simulink model "DAB_Data_Generate_v2"  (R2021b)
settings: Solver=FixedStepAuto  StartTime=0.0  StopTime=1  FixedStep=1e-6  MaxStep=1e-4  RelTol=1e-3
values from neighbouring files (symbols this model uses):
  f = 50e3    (= 50000)    [DAB_Data_Generation.m]
  N_pri = 1000    [DAB_Data_Generation.m]
  N_sec = 1000    [DAB_Data_Generation.m]
  Vin = 400    [DAB_Data_Generation.m]
undefined symbols (not defined in the file or in its folder): D0, D1, D2, P
libraries: spsOnDelayLib x8, spsIGBTDiodeLib x8, spsVoltageMeasurementLib x4, spsCurrentMeasurementLib x4, spsSeriesRLCBranchLib x3, spsDCVoltageSourceLib x1, spsLinearTransformerLib x1, spsMeanLib x1, spsRMSLib x1, spspowerguiLib x1
settings Model: Creator=mluser  LastModifiedBy=varat
settings SolverCC: AlgebraicLoopSolver=TrustRegion
settings DebuggingCC: ArithmeticOperatorsInVariantConditions=warning
settings SFSimCC: CustomCodeUndefinedFunction=UseInterfaceOnly

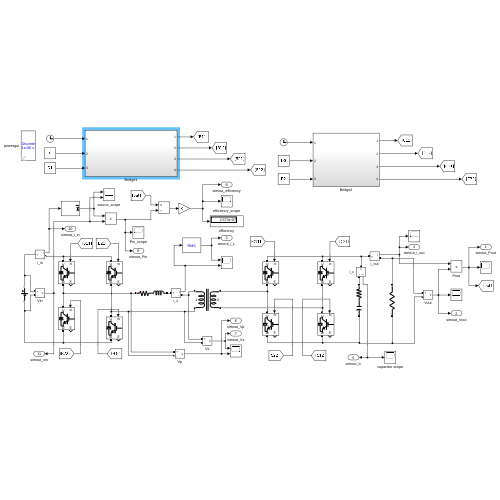
[thumbnail: Simulink's stored preview of the top-level diagram]
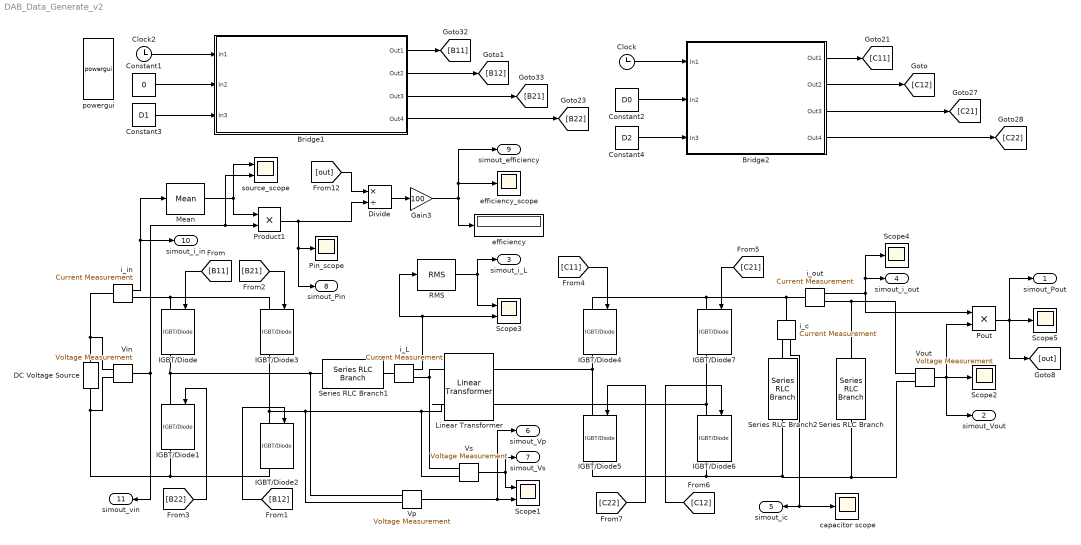
== system DAB_Data_Generate_v2 ==
  Bridge1 : Subsystem
  Bridge2 : Subsystem
  Clock : Clock
  Clock2 : Clock
  Constant1 : Constant  Value=0
  Constant2 : Constant  Value=D0
  Constant3 : Constant  Value=D1
  Constant4 : Constant  Value=D2
  DC Voltage Source : spsDCVoltageSourceLib/DC Voltage Source  Amplitude=Vin  Measurements=None
  Divide : Product  Inputs=*/
  Gain3 : Gain  Gain=100
  IGBT/Diode{,1..7} (8 alike) : spsIGBTDiodeLib/IGBT//Diode  Ron=1e-4  Rs=1e5  Cs=inf  Measurements=on
  Linear Transformer : spsLinearTransformerLib/Linear Transformer  UNITS=SI  NominalPower=[300e3 50000 ]  winding1=[N_pri 0 0]  winding2=[N_sec 0 0]  ThreeWindings=off  winding3=[3.15e+05 793.8 0.10107]  RmLm=[2e+12 3.9789e+08]  Measurements=None  DataType=on
  Mean : spsMeanLib/Mean  Freq=50000  Vinit=0  Ts=0
  Pin_scope : Scope
  Pout : Product
  Product1 : Product
  RMS : spsRMSLib/RMS  TrueRMS=on  Freq=50000  RMSInit=0  Ts=0
  Scope1 : Scope  NumInputPorts=2
  Scope2 : Scope
  Scope3 : Scope  NumInputPorts=2
  Scope4 : Scope
  Scope5 : Scope
  Series RLC Branch : spsSeriesRLCBranchLib/Series RLC Branch  LConnTagsString=__new0  RConnTagsString=__new0  BranchType=R  Resistance=(400*400)/P  Inductance=1e-3  SetiL0=off  InitialCurrent=0  Capacitance=1e-6  Setx0=off  InitialVoltage=0  Measurements=None
  Series RLC Branch1 : spsSeriesRLCBranchLib/Series RLC Branch  LConnTagsString=__new0  RConnTagsString=__new0  BranchType=RL  Resistance=0  Inductance=2.42649e-6  SetiL0=off  InitialCurrent=0  Capacitance=1e-6  Setx0=off  InitialVoltage=0  Measurements=None
  Series RLC Branch2 : spsSeriesRLCBranchLib/Series RLC Branch  LConnTagsString=__new0  RConnTagsString=__new0  BranchType=RC  Resistance=0  Inductance=1e-3  SetiL0=off  InitialCurrent=0  Capacitance=10e-3  Setx0=off  InitialVoltage=0  Measurements=None
  Vin : spsVoltageMeasurementLib/Voltage Measurement  PhasorSimulation=off  OutputType=Complex  PSBequivalent=0
  Vout : spsVoltageMeasurementLib/Voltage Measurement  PhasorSimulation=off  OutputType=Complex  PSBequivalent=0
  Vp : spsVoltageMeasurementLib/Voltage Measurement  PhasorSimulation=off  OutputType=Complex  PSBequivalent=0
  Vs : spsVoltageMeasurementLib/Voltage Measurement  PhasorSimulation=off  OutputType=Complex  PSBequivalent=0
  capacitor scope : Scope
  efficiency : Display
  efficiency_scope : Scope
  i_L : spsCurrentMeasurementLib/Current Measurement  PhasorSimulation=off  OutputType=Complex  PSBequivalent=0
  i_c : spsCurrentMeasurementLib/Current Measurement  PhasorSimulation=off  OutputType=Complex  PSBequivalent=0
  i_in : spsCurrentMeasurementLib/Current Measurement  PhasorSimulation=off  OutputType=Complex  PSBequivalent=0
  i_out : spsCurrentMeasurementLib/Current Measurement  PhasorSimulation=off  OutputType=Complex  PSBequivalent=0
  powergui : spspowerguiLib/powergui  Priority=1  SimulationMode=Discrete  SampleTime=1e-6  frequency=60  Iterations=50  frequencyindice=0  Pbase=100e6  ErrMax=1e-4  UnitsV=kV  UnitsW=MW  buscounter=0  FunctionMessages=off  echomessages=off  EnableUseOfTLC=off  CurrentSourceSwitches=off  DisableSnubberDevices=off  DisableRonSwitches=off  DisableVfSwitches=off  DisplayEquations=off  AutomaticDiscreteSolvers=off  SolverType=Tustin/Backward Euler (TBE)  Interpol=off  ExternalGateDelay=off  methode=off  Ts=100  x0status=blocks  SPID=off  SwTol=0  HookPort=off  NonlinearTolerance=1e-4  nMaxIteration=100  ContinueOnMaxIteration=off  RestoreLinks=warning  ResistiveCurrentMeasurement=off  Frange=[0:2:500]  Ylog=off  Xlog=on  ShowGrid=off  save=off  variable=ZData  structure=0  ZoomFFT=off  StartTime=0.0  cycles=1  DisplayStyle=1  fundamental=60  FreqAxis=off  MaxFrequency=1000  frequencyindicesteady=1  RmsSteady=1  display=off
  source_scope : Scope  NumInputPorts=2
  simout_Pout : Outport
  simout_Vout : Outport  Port=2
  simout_i_L : Outport  Port=3
  simout_i_out : Outport  Port=4
  simout_ic : Outport  Port=5
  simout_Vp : Outport  Port=6
  simout_Vs : Outport  Port=7
  simout_Pin : Outport  Port=8
  simout_efficiency : Outport  Port=9
  simout_i_in : Outport  Port=10
  simout_vin : Outport  Port=11
  wires:
  RMS/1 -> simout_i_L/1, Scope3/1
  [C12] -> IGBT/Diode6/1
  Vin/1 -> simout_vin/1, source_scope/2, Product1/2
  [C11] -> IGBT/Diode4/1
  [B11] -> IGBT/Diode/1
  Mean/1 -> source_scope/1, Product1/1
  [C21] -> IGBT/Diode7/1
  [out] -> Divide/1
  [B21] -> IGBT/Diode3/1
  [B22] -> IGBT/Diode1/1
  [C22] -> IGBT/Diode5/1
  Gain3/1 -> simout_efficiency/1, efficiency_scope/1, efficiency/1
  Product1/1 -> simout_Pin/1, Pin_scope/1, Divide/2
  i_out/1 -> Scope4/1, simout_i_out/1, Pout/1
  Vout/1 -> simout_Vout/1, Scope2/1, Pout/2
  Divide/1 -> Gain3/1
  Pout/1 -> simout_Pout/1, [out], Scope5/1
  i_L/1 -> Scope3/2, RMS/1
  [B12] -> IGBT/Diode2/1
  Bridge2/1(Out1) -> [C11]
  Constant1/1 -> Bridge1/2(In2)
  Clock2/1 -> Bridge1/1(In1)
  Constant2/1 -> Bridge2/2(In2)
  Bridge1/3(Out3) -> [B21]
  Clock/1 -> Bridge2/1(In1)
  Bridge2/4(Out4) -> [C22]
  Bridge1/2(Out2) -> [B12]
  Bridge2/3(Out3) -> [C21]
  Bridge1/1(Out1) -> [B11]
  Bridge2/2(Out2) -> [C12]
  Bridge1/4(Out4) -> [B22]
  Constant4/1 -> Bridge2/3(In3)
  Constant3/1 -> Bridge1/3(In3)
  Vs/1 -> Scope1/1, simout_Vs/1
  Vp/1 -> simout_Vp/1, Scope1/2
  i_c/1 -> simout_ic/1, capacitor scope/1
  i_in/1 -> simout_i_in/1, Mean/1
  connections:
  Vp/LConn1 -- Series RLC Branch1/LConn1 -- IGBT/Diode1/LConn1 -- IGBT/Diode/RConn1
  Linear Transformer/LConn1 -- Vs/LConn1 -- i_L/RConn1
  Vp/LConn2 -- Vs/LConn2 -- Linear Transformer/LConn2 -- IGBT/Diode3/RConn1 -- IGBT/Diode2/LConn1
  i_out/RConn1 -- Vout/LConn1 -- Series RLC Branch/LConn1
  Linear Transformer/RConn1 -- IGBT/Diode5/LConn1 -- IGBT/Diode4/RConn1
  IGBT/Diode5/RConn1 -- IGBT/Diode6/RConn1 -- Series RLC Branch2/RConn1 -- Vout/LConn2 -- Series RLC Branch/RConn1
  i_in/RConn1 -- IGBT/Diode3/LConn1 -- IGBT/Diode/LConn1
  i_out/LConn1 -- IGBT/Diode4/LConn1 -- IGBT/Diode7/LConn1 -- i_c/LConn1
  Linear Transformer/RConn2 -- IGBT/Diode7/RConn1 -- IGBT/Diode6/LConn1
  IGBT/Diode2/RConn1 -- IGBT/Diode1/RConn1 -- Vin/LConn2 -- DC Voltage Source/LConn1
  i_in/LConn1 -- Vin/LConn1 -- DC Voltage Source/RConn1
  i_L/LConn1 -- Series RLC Branch1/RConn1
  Series RLC Branch2/LConn1 -- i_c/RConn1

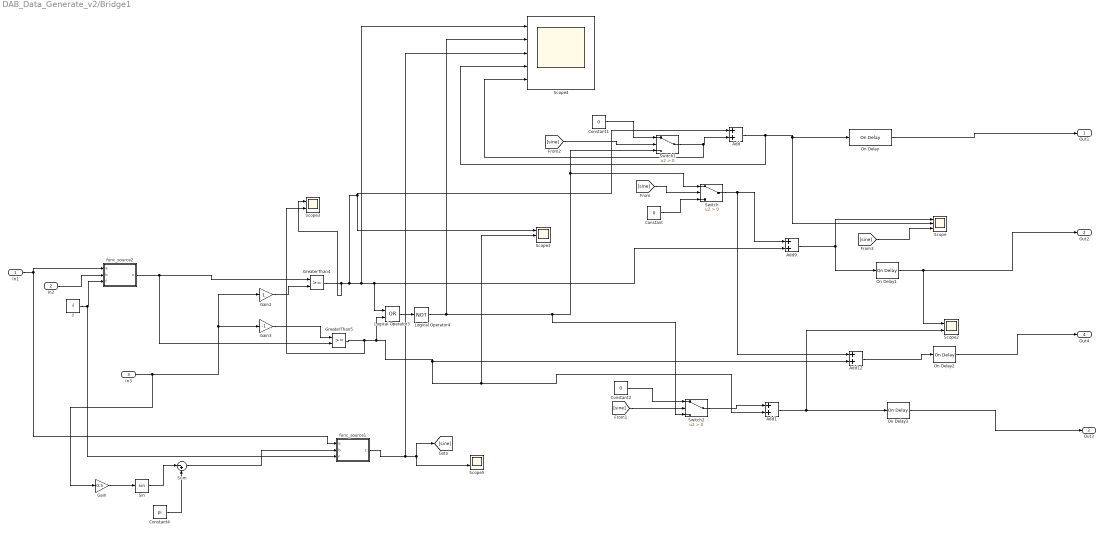
== system DAB_Data_Generate_v2/Bridge1 ==
  In1 : Inport
  In2 : Inport  Port=2
  In3 : Inport  Port=3
  Add{,1,9,12} (4 alike) : Sum
  Constant : Constant  Value=0
  Constant1 : Constant  Value=0
  Constant2 : Constant  Value=0
  Constant4 : Constant  Value=pi
  Gain : Gain  Gain=0.5
  Gain2 : Gain
  Gain3 : Gain  Gain=-1
  GreaterThan4 : RelationalOperator  OutDataTypeStr=boolean  RndMeth=Simplest
  GreaterThan5 : RelationalOperator  OutDataTypeStr=boolean  RndMeth=Simplest
  Logical Operator3 : Logic  Operator=OR  AllPortsSameDT=off  OutDataTypeStr=boolean
  Logical Operator4 : Logic  Operator=NOT  AllPortsSameDT=off  OutDataTypeStr=boolean
  On Delay{,1..3} (4 alike) : spsOnDelayLib/On Delay  DelayType=On delay  delay=0  ic=0  Ts=0
      settings: SourceProductBaseCode=PS
  Scope : Scope  NumInputPorts=3
  Scope1 : Scope  NumInputPorts=3
  Scope2 : Scope  NumInputPorts=2
  Scope3 : Scope  NumInputPorts=2
  Scope4 : Scope  NumInputPorts=5
  Scope5 : Scope  NumInputPorts=2
  Sin : Trigonometry
  Sum : Sum  Inputs=|-+
  Switch : Switch  Criteria=u2 > Threshold
  Switch1 : Switch  Criteria=u2 > Threshold
  Switch2 : Switch  Criteria=u2 > Threshold
  f : Constant  Value=f
  func_source1 : MATLAB Function  TreatAsAtomicUnit=on
  func_source2 : MATLAB Function  TreatAsAtomicUnit=on
  Out1 : Outport  VectorParamsAs1DForOutWhenUnconnected=off
  Out2 : Outport  Port=2  VectorParamsAs1DForOutWhenUnconnected=off
  Out3 : Outport  Port=3  VectorParamsAs1DForOutWhenUnconnected=off
  Out4 : Outport  Port=4  VectorParamsAs1DForOutWhenUnconnected=off
  wires:
  [sine] -> Scope/3
  Gain2/1 -> GreaterThan4/2
  Add/1 -> Scope4/4, Scope/2, On Delay/1
  Add1/1 -> Scope2/2, On Delay3/1
  Add9/1 -> On Delay1/1, Scope/1
  On Delay/1 -> Out1/1
  Add12/1 -> On Delay2/1
  Switch/1 -> Add12/1, Add9/1
  Logical Operator3/1 -> Logical Operator4/1
  Switch2/1 -> Add1/1
  [sine] -> Switch/2
  [sine] -> Switch1/2
  GreaterThan5/1 -> Scope3/2, Scope1/2, Add1/2, Add12/2, Logical Operator3/2
  Logical Operator4/1 -> Scope4/2, Switch2/3, Switch/1, Switch1/3
  Gain3/1 -> GreaterThan5/1
  In3/1 -> Gain/1, Gain3/1, Gain2/1
  [sine] -> Switch2/2
  On Delay3/1 -> Out3/1
  On Delay2/1 -> Out4/1
  On Delay1/1 -> Out2/1, Scope2/1
  GreaterThan4/1 -> Scope3/1, Add/1, Scope1/1, Scope4/1, Add9/2, Logical Operator3/1
  In1/1 -> func_source1/1(a), func_source2/1(a)
  Switch1/1 -> Scope4/5, Add/2
  func_source1/1(z) -> Scope4/3, [sine], Scope5/2
  Sum/1 -> func_source1/2(b)
  func_source2/1(z) -> GreaterThan5/2, GreaterThan4/1
  In2/1 -> func_source2/2(b)
  Constant1/1 -> Switch1/1
  Constant/1 -> Switch/3
  Constant2/1 -> Switch2/1
  Gain/1 -> Sin/1
  Constant4/1 -> Sum/2
  Sin/1 -> Sum/1
  f/1 -> func_source1/3(f), func_source2/3(f)

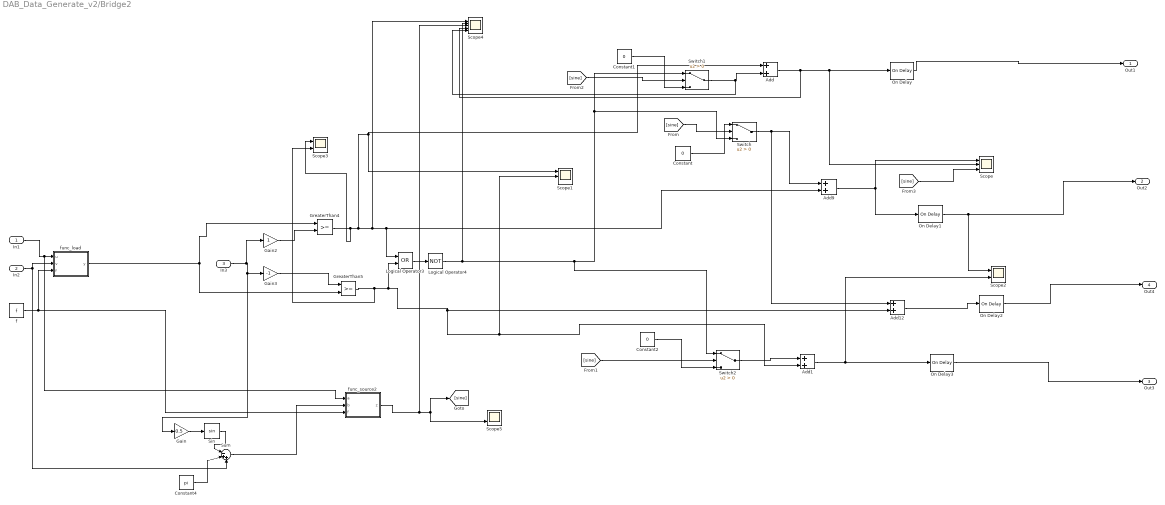
== system DAB_Data_Generate_v2/Bridge2 ==
  In1 : Inport
  In2 : Inport  Port=2
  In3 : Inport  Port=3
  Add{,1,9,12} (4 alike) : Sum
  Constant : Constant  Value=0
  Constant1 : Constant  Value=0
  Constant2 : Constant  Value=0
  Constant4 : Constant  Value=pi
  Gain : Gain  Gain=0.5
  Gain2 : Gain
  Gain3 : Gain  Gain=-1
  GreaterThan4 : RelationalOperator  OutDataTypeStr=boolean  RndMeth=Simplest
  GreaterThan5 : RelationalOperator  OutDataTypeStr=boolean  RndMeth=Simplest
  Logical Operator3 : Logic  Operator=OR  AllPortsSameDT=off  OutDataTypeStr=boolean
  Logical Operator4 : Logic  Operator=NOT  AllPortsSameDT=off  OutDataTypeStr=boolean
  On Delay{,1..3} (4 alike) : spsOnDelayLib/On Delay  DelayType=On delay  delay=0  ic=0  Ts=0
      settings: SourceProductBaseCode=PS
  Scope : Scope  NumInputPorts=3
  Scope1 : Scope  NumInputPorts=3
  Scope2 : Scope  NumInputPorts=2
  Scope3 : Scope  NumInputPorts=2
  Scope4 : Scope  NumInputPorts=5
  Scope5 : Scope  NumInputPorts=2
  Sin : Trigonometry
  Sum : Sum  Inputs=|-++
  Switch : Switch  Criteria=u2 > Threshold
  Switch1 : Switch  Criteria=u2 > Threshold
  Switch2 : Switch  Criteria=u2 > Threshold
  f : Constant  Value=f
  func_load : MATLAB Function  TreatAsAtomicUnit=on
  func_source2 : MATLAB Function  TreatAsAtomicUnit=on
  Out1 : Outport  VectorParamsAs1DForOutWhenUnconnected=off
  Out2 : Outport  Port=2  VectorParamsAs1DForOutWhenUnconnected=off
  Out3 : Outport  Port=3  VectorParamsAs1DForOutWhenUnconnected=off
  Out4 : Outport  Port=4  VectorParamsAs1DForOutWhenUnconnected=off
  wires:
  [sine] -> Scope/3
  Gain2/1 -> GreaterThan4/2
  Add/1 -> Scope4/4, On Delay/1, Scope/2
  Add1/1 -> Scope2/2, On Delay3/1
  Add9/1 -> On Delay1/1, Scope/1
  On Delay/1 -> Out1/1
  Add12/1 -> On Delay2/1
  Switch/1 -> Add12/1, Add9/1
  Logical Operator3/1 -> Logical Operator4/1
  Switch2/1 -> Add1/1
  [sine] -> Switch/2
  [sine] -> Switch1/2
  GreaterThan5/1 -> Scope3/2, Scope1/2, Add1/2, Add12/2, Logical Operator3/2
  Logical Operator4/1 -> Scope4/2, Switch2/1, Switch/3, Switch1/1
  Gain3/1 -> GreaterThan5/1
  func_load/1(y) -> GreaterThan5/2, GreaterThan4/1
  [sine] -> Switch2/2
  On Delay3/1 -> Out3/1
  On Delay2/1 -> Out4/1
  On Delay1/1 -> Out2/1, Scope2/1
  GreaterThan4/1 -> Scope3/1, Add/1, Scope1/1, Scope4/1, Add9/2, Logical Operator3/1
  In1/1 -> func_source2/1(a), func_load/1(u)
  Switch1/1 -> Scope4/5, Add/2
  func_source2/1(z) -> Scope4/3, [sine], Scope5/2
  Sum/1 -> func_source2/2(b)
  In2/1 -> Sum/3, func_load/2(v)
  Constant1/1 -> Switch1/3
  Constant2/1 -> Switch2/3
  Constant/1 -> Switch/1
  Constant4/1 -> Sum/2
  Gain/1 -> Sin/1
  In3/1 -> Gain2/1, Gain/1, Gain3/1
  Sin/1 -> Sum/1
  f/1 -> func_source2/3(f), func_load/3(f)

== matlab function DAB_Data_Generate_v2/Bridge1/func_source2 ==
  data: a input; z output; b input; f input
function z = fcn(a,b, f)
%#codegen

z = sin(2*pi*f*a - b);
end

== matlab function DAB_Data_Generate_v2/Bridge2/func_source2 ==
  data: a input; z output; b input; f input
function z = fcn(a,b,f)
%#codegen

z = sin(2*pi*f*a - b);
end

== matlab function DAB_Data_Generate_v2/Bridge1/func_source1 ==
  data: a input; z output; b input; f input
function z = fcn(a,b,f)
%#codegen

z = sin(2*pi*f*a - b);
end

== matlab function DAB_Data_Generate_v2/Bridge2/func_load ==
  data: u input; y output; v input; f input
function y = fcn(u,v,f)
%#codegen

y = sin(2*pi*f*u - v );
end
